simulink model "yawDamperCheckDesign1"  (R2018b)
settings: Solver=VariableStepAuto  StartTime=0.0  StopTime=50  RelTol=1e-3
undefined symbols (not defined in the file): sigbuilder_block
libraries: cstblocks x2, simulink_extras x2, dspsrcs4 x1
settings Model: Creator=engmh  LastModifiedBy=OWNER
settings DataIOCC: ReturnWorkspaceOutputs=on
settings DebuggingCC: LibraryContextMissingDiagnostic=none  SFMachineParentedDataDiag=error

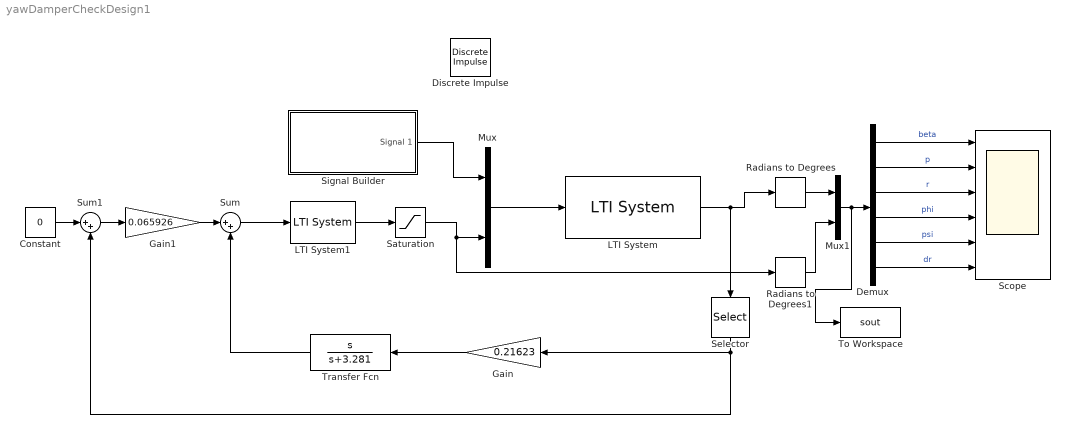
== system yawDamperCheckDesign1 ==
  Constant : Constant  Value=0
  Demux : Demux  Outputs=6
  Discrete Impulse : dspsrcs4/Discrete  Impulse  Delay=0  SampleTime=1  FrameSample=1  OutputFrames=off  dataType=double  isSigned=on  wordLen=16  udDataType=sfix(16)  fracBitsMode=Best precision  numFracBits=15  OutDataTypeStr=double  LastOutDataTypeStr=double
  Gain : Gain  Gain=0.21623
  Gain1 : Gain  Gain=0.065926
  LTI System : cstblocks/LTI System  sys=LatSS  IC=[]
  LTI System1 : cstblocks/LTI System  sys=servo  IC=[]
  Mux : Mux  Inputs=2
  Mux1 : Mux  Inputs=2
  Radians to Degrees : simulink_extras/Transformations/Radians to Degrees
  Radians to Degrees1 : simulink_extras/Transformations/Radians to Degrees
  Saturation : Saturate  UpperLimit=15*pi/180  LowerLimit=-15*pi/180
  Scope : Scope  NumInputPorts=6
  Selector : Selector  InputPortWidth=5  IndexOptions=Index vector (dialog)  Indices=[3]  OutputSizes=1
  Signal Builder : Subsystem  Tag=STV Subsys  LoadFcn=sigbuilder_block('load');  StartFcn=sigbuilder_block('start');  StopFcn=sigbuilder_block('stop');  ClipboardFcn=sigbuilder_block('clipboard');  mask(Sigbuilder block){tuvar=[0:10]}
      mask help: Simulink:masks:SigbuilderBlock_MD
      mask init:
      | if ~strcmp(get_param(bdroot(gcbh),'SimulationStatus'),'stopped') tuvar = sigbuilder_block('maskInit'); end
      settings: CopyFcn=sigbuilder_block('copy');  DeleteFcn=sigbuilder_block('delete');  ModelCloseFcn=sigbuilder_block('modelClose');  PreSaveFcn=sigbuilder_block('preSave');  PauseFcn=sigbuilder_block('pause');  ContinueFcn=sigbuilder_block('continue');  NameChangeFcn=sigbuilder_block('namechange');  OpenFcn=sigbuilder_block('open',[64.2 261 583.05 372.75 ]);  CloseFcn=sigbuilder_block('close');
      mask Display: plot(0, 0, 100, 100,[2, 2, 32, 32, 2], [68, 8, 8, 68, 68],[32, 2], [38, 38], [32, 19, 2],[53, 60, 44], [32, 17, 17, 2],[16, 16, 31, 31]);txt = getActiveGroup(gcbh);text(2, 100, txt,'verticalAlignment', 'top');
  Sum : Sum  Inputs=|++
  Sum1 : Sum  Inputs=|++
  To Workspace : ToWorkspace  VariableName=sout  SaveFormat=Timeseries  SampleTime=-1
  Transfer Fcn : TransferFcn  Numerator=[1 0]  Denominator=[1 3.281]
  wires:
  Gain/1 -> Transfer Fcn/1
  LTI System/1 -> Radians to Degrees/1, Selector/1
  Selector/1 -> Sum1/2, Gain/1
  Transfer Fcn/1 -> Sum/2
  Constant/1 -> Sum1/1
  Sum/1 -> LTI System1/1
  LTI System1/1 -> Saturation/1
  Mux/1 -> LTI System/1
  Demux/1 -> Scope/1  "beta"
  Demux/2 -> Scope/2  "p"
  Demux/3 -> Scope/3  "r"
  Demux/4 -> Scope/4  "phi"
  Demux/5 -> Scope/5  "psi"
  Mux1/1 -> To Workspace/1, Demux/1
  Radians to Degrees/1 -> Mux1/1
  Radians to Degrees1/1 -> Mux1/2
  Demux/6 -> Scope/6  "dr"
  Saturation/1 -> Radians to Degrees1/1, Mux/2
  Signal Builder/1(Signal 1) -> Mux/1
  Sum1/1 -> Gain1/1
  Gain1/1 -> Sum/1

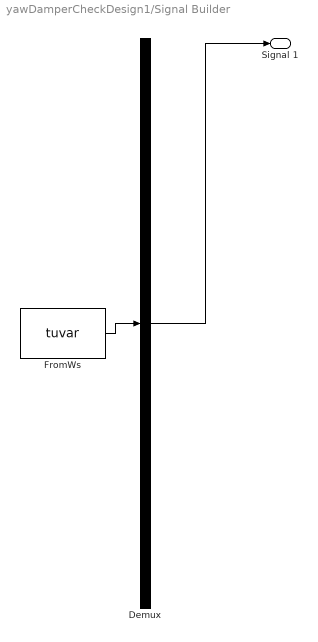
== system yawDamperCheckDesign1/Signal Builder ==
  Demux : Demux  Tag=STV Demux  Outputs=1
  FromWs : FromWorkspace  Tag=STV FromWs  VariableName=tuvar  SampleTime=0
      SigBuilderData=|
      | common.afterFinalStr = 'Extrapolate'
      | common.sampleTime = 0
      | dataSet.timeRange = [0 10]
      | dataSet.name = 'Group 1'
      | sbobj.Groups.Name = 'Group 1'
      | sbobj.Groups.Signals.Name = 'Signal 1'
      | sbobj.Groups.Signals.XData = [0 0.98 0.98 1.98 1.98 10]
      | sbobj.Groups.Signals.YData = [0 0 0.1005 0.1005 0 0]
  Signal 1 : Outport  Tag=STV Outport  VectorParamsAs1DForOutWhenUnconnected=on
  wires:
  Demux/1 -> Signal 1/1
  FromWs/1 -> Demux/1
